simulink model "Expriment_Pose"  (R2014a)
settings: Solver=FixedStepDiscrete  SolverMode=SingleTasking  StartTime=0.0  StopTime=inf  FixedStep=0.01  RelTol=1e-3
PostLoadFcn:
  | h_RPStest = RPStest;
model workspace (MAT data in the model file):
  gtest = 0
undefined symbols (not defined in the file or in its folder): avert, avert_freq_factor, avert_gaze_dirs_chance, avert_gaze_duration_factor, avert_head_frequency_factor, avert_head_speed, BML, BML1, BML2, bmlsL, bmlsM, bodyBusyFlag, clock, emotion_amount_factor, faceBusyFlag, fileID, GAZE_WIN, gazing, mut_freq_factor, mutual_gaze_duration_factor, P, pose_cat_chance, pose_chanc_factor, pose_chance_factor, pose_frequency_factor, pose_lean, pose_lean_flag, pose_speed, pose_twitch, pr, serial, STATE_BEFORE, STATE_GO, STATE_OVER, STATE_READY, Stateflow
libraries: simulink x24, instrumentlib x6, lib_affectiveChar_behavior x2, realtime_pacer_lib x2, lib_affectiveChar_input x1
(part 6 of 7)

== stateflow chart Expriment_Pose/CharacterControl/idlePose_Controller ==
  note: PERSONALITY:
      | -HN: self-touching and object manipulations, non-fluencies rigid posture and minimization of random movements, erect shoulder, cross legs Lean forward tenser
      | -LN:Lean backward reclining, head lean sideway or down
      | -High arousal: self and object adaptors, body tension and random trunk
      | For more info check Burgoon and Koper, 1984.
  note: -Ekman categorized hand poses to Emblems(e.g. hand shrug for helplessness or inability ; thumbs up), illustrators, Regulators, POINTS, Adaptors (self, alter-directed), spontaneousgests, attention-based gests
      | -Picking or squeezing part of the body is aggression against the self or aggression towards others temporarily displaced onto the self;
      | -covering the eye with a hand is relevant to preventing input, avoiding being seen, and shame
      | For more infor refer to Ekman (1972) Hand Movements.
  note: continously unpdate values based on change in valence-arousal
  note: The higher BOREDOMT (treshold), the lower chance of bored pose.
  note: Logically, personality parameters should only get calculated once. Since, here we change the personality dynamically during simulation,we calculate it in each loop.
  note: Problems with priortizing behaviors:
      |     1) When personality change, we want a few adjustments to happen e.g. agent's lean pose changes. The problem is system detects the change and set the flag to 1 and then again goes back to 0. If we dont check in stateflow exactly at that time we dont detect the change. that's why we need another flag that keeps the change till we do the personality based adjustment in behavior.After doing the adjustment we set that flag to zero.
      |     2) We can not use this for tracking if the body is busy at the time. When there is environmnet change agent reacts either by face or body (faceBusyFlag and bodyBusyFlag). We want to stop sending idle BML when they are busy. We need to check if flag is 1 excatly when we want to send the idle body or gaze BML.(if its a few milisec after or before it may not be busy. That's why we need attendChange module to set the flag to 1 for 10 sec after bodyBusy or faceBusy to avoid generating idle behavior in that period.
      |     3)problem also occures when the agent is at the middle of an idle pose/avert and needs to do interactive pose. It causes averted head+smile etc.
  note: Brebner pointed out that frequency of hand movements/gestures was positively correlated with Extraversion [9].
      | Brebner, J. 1985. Personality theory and movement. In B.D. Kirkcaldy (Ed.), Individual differences in movement (pp.
      | 27-41). Lancaster, England: MTP Press Limited.
  note: Riggio suggested that extraverts change their posture more often.
      | Riggio, R., Friedman, H. 1986. Impression formation: The
      | role of expressive behavior. In Journal of Personality and
      | Social Psychology 50(2), 421-427
  state idlePoseGenerate [parallel]
    settings: executionOrder=1
    state stateInit
      entry:STATE_OVER=3;STATE_BEFORE=4;pose_lean_flag=0;
      STATE_READY=7;STATE_GO=1;gameState= 14;
      n=encStr2Arr(' ');bmlsL=[n n n n n];newBmlsL=[n n n n n];
      pose_frequency_factor=20;pose_chance_factor=1;pose_cat_chance=70;
      pose_lean=10; pose_speed=1;pose_lean_flag=0;pose_twitch=0;
    state leanChange
      entry:  pose_lean_flag=0;
      [P,BMLM]=weightshiftTable(pose_lean) ;
      newBmlsM=insertQueue(bmlsM,BMLM);
      bmlsM=newBmlsM;
    state stateRandomPose
      entry: randSlowPose=randArray(:,11);%(1,5)
      interest=BOREDOM_THRESHOLD-boredom;interest=1;
    state stateExtrovertPoseChance
      entry: randPoseChance=randi([0,round(interest*randSlowPose/pose_chance_factor)]);
    note: SLOW
    note: FAST
    note: else
    note: else
    state poseCategoryChance1
      entry: randPR=randArray(:,20);
    state poseCategoryChance2
      entry: randPR=randArray(:,20);
    state poseCategoryChance
      entry: randPR=randArray(:,20);
    note: else
    note: else
    state selfAdaptorPoseCategory
      entry:pose_type=selfAdaptorTypeTable(pose_speed, pose_twitch);
      [P,BMLl]=selfAdaptorTable(randArray(:,pose_type)) ;
      newBmlsL=insertQueueLow(bmlsL,BMLl);
      bmlsL=newBmlsL;%disp(decArr2Str(BMLl));
    state weightshiftPoseCategory
      entry:pose_type=weightShiftTypeTable(pose_speed);
      [P,BMLl]= weightshiftTable(randArray(:,pose_type));
      newBmlsL=insertQueueLow(bmlsL,BMLl);
      bmlsL=newBmlsL;
    (default) -> stateInit
    stateInit -> stateRandomPose
    leanChange -> stateRandomPose : after(1,secs)
    stateRandomPose -> leanChange [order 1] : [pose_lean_flag==1]
    (junction 2) -> stateRandomPose [order 2]
    weightshiftPoseCategory -> stateRandomPose : after(pose_frequency_factor,secs)
    (junction 425) -> stateRandomPose [order 2]
    stateRandomPose -> stateExtrovertPoseChance [order 2]
    selfAdaptorPoseCategory -> stateRandomPose : after(pose_frequency_factor,secs)
    (junction 169) -> stateRandomPose [order 2]
    stateExtrovertPoseChance -> (junction 2) [order 2] : [pose_speed==2]
    stateExtrovertPoseChance -> (junction 425) [order 3] : [pose_speed==1]
    stateExtrovertPoseChance -> (junction 169) [order 1] : [pose_speed==3]
    (junction 425) -> poseCategoryChance2 [order 1] : [[randPoseChance==1]&[ gameState~= STATE_GO]&[ gameState~= STATE_READY]]
    (junction 2) -> poseCategoryChance1 [order 1] : [[randPoseChance==1]&[ gameState~= STATE_GO]&[ gameState~= STATE_READY]]
    (junction 169) -> poseCategoryChance [order 1] : [[randPoseChance==1]&[ gameState~= STATE_GO]&[ gameState~= STATE_READY]]
    poseCategoryChance2 -> poseCategoryChance2 [order 2]
    poseCategoryChance1 -> poseCategoryChance1 [order 2]
    poseCategoryChance -> poseCategoryChance [order 2]
    poseCategoryChance1 -> (junction 344) [order 1] : [bodyBusyFlag~=1]
    poseCategoryChance2 -> (junction 431) [order 1] : [bodyBusyFlag~=1]
    poseCategoryChance -> (junction 340) [order 1] : [bodyBusyFlag~=1]
    (junction 340) -> (junction 212) [order 1] : [randPR<=pose_cat_chance]
    (junction 431) -> (junction 211) [order 2] : [randPR>pose_cat_chance]
    (junction 431) -> (junction 212) [order 1] : [randPR<=pose_cat_chance]
    (junction 344) -> (junction 211) [order 1] : [randPR<=pose_cat_chance]
    (junction 340) -> (junction 211) [order 2] : [randPR>pose_cat_chance ]
    (junction 344) -> (junction 212) [order 2] : [randPR>pose_cat_chance]
    (junction 212) -> weightshiftPoseCategory
    (junction 211) -> selfAdaptorPoseCategory
  note: randSlowPose=randi(1,6)
  note: D10 for animation 8 which is hand on waist may not work with wave etc. Too long!
  note: McNeill's gesture space sectors: the performance space in front of an actor is divided into three gesture space sections: Center-Center (CC), Center (C), and Periphery (P). CC is the central section directly in front of the chest, while subsequent sections (C and P) form spatial layers spreading outwards. low-warmth-low-competence performance consists of gestures mostly in the lower, center P region, while high-warmth-high-competence focuses mostly in the CC and C regions.
  note: LEHN error : more weight shidt
  data: bmlID function_input double; pr function_output double size=1; poseBML function_output double size=[1000,1]; bmlID function_input double; pr function_output double size=1; poseBML function_output double size=[1000,1]; pr function_output double size=1; bmlID function_input double; poseBML function_output double size=[1000,1]; poseSpeed function_input double size=1; shiftType function_output double size=1; poseSpeed function_input double size=1; poseTwitch function_input double size=1; poseType function_output double size=1; bmls function_input double size=[1000,5]; myBML function_input double size=[1000,1]; newBmls function_output double size=[1000,5]; bmls function_input double size=[1000,5]; myBML function_input double size=[1000,1]; newBmls function_output double size=[1000,5]; boredom data_store_memory size=2; BOREDOM_THRESHOLD data_store_memory size=2; randSlowPose data_store_memory size=2; interest data_store_memory size=2; gameState output double size=1; randPoseChance data_store_memory size=1; STATE_OVER data_store_memory size=2; STATE_BEFORE data_store_memory size=2; STATE_READY data_store_memory size=2; inA input double size=1; inE input double size=1; HAPPY data_store_memory size=1 =4; SAD data_store_memory size=1 =4; CONTEMPT data_store_memory size=1 =4; BORED data_store_memory size=1 =4; FRUST data_store_memory size=1 =4; FEAR data_store_memory size=1 =4; IDLE data_store_memory size=1 =4; EXCITE data_store_memory size=1 =4; BML data_store_memory size=[256,1]; P data_store_memory; fileID data_store_memory; STATE_GO data_store_memory; bodyBusyFlag data_store_memory; BMLM local double size=[1000,1]; newBmlsL local double size=[1000,5]; bmlsL data_store_memory; n local; randArray input double size=[1,25]; personality input double size=1; randPR local; pPoseChance local; poseFreq local; leanPose local; inV input double size=1; pPoseChanceP local; poseFreqP local; pCatChance local; catChance local; personalityChange input boolean size=1; bmlsM data_store_memory; BMLl local double size=[1000,1]; newBmlsM local double size=[1000,5]; pChangeFlag local; faceBusyFlag data_store_memory; poseArray input double size=[1, 6]; pose_speed data_store_memory; pose_lean_flag data_store_memory; pose_lean data_store_memory; pose_frequency_factor data_store_memory; pose_chance_factor data_store_memory; pose_cat_chance data_store_memory; pose_change_flag data_store_memory; pose_type local; pose_twitch data_store_memory
  events: secs input RISING_EDGE_EVENT
  function [pr,poseBML]=selfAdaptorTableBilly(bmlID):
    | function [pr,poseBML]=selfAdaptorTableBilly(bmlID)
    | 
    | aVarTruthTableCondition_1 = false;
    | aVarTruthTableCondition_2 = false;
    | aVarTruthTableCondition_3 = false;
    | aVarTruthTableCondition_4 = false;
    | aVarTruthTableCondition_5 = false;
    | aVarTruthTableCondition_6 = false;
    | aVarTruthTableCondition_7 = false;
    | aVarTruthTableCondition_8 = false;
    | aVarTruthTableCondition_9 = false;
    | aVarTruthTableCondition_10 = false;
    | aVarTruthTableCondition_11 = false;
    | aVarTruthTableCondition_12 = false;
    | aVarTruthTableCondition_13 = false;
    | aVarTruthTableCondition_14 = false;
    | aVarTruthTableCondition_15 = false;
    | aVarTruthTableCondition_16 = false;
    | aVarTruthTableCondition_17 = false;
    | aVarTruthTableCondition_18 = false;
    | aVarTruthTableCondition_19 = false;
    | aVarTruthTableCondition_20 = false;
    | 
    | 
    | 
    | aVarTruthTableCondition_1 = logical(bmlID==1);
    | 
    | 
    | aVarTruthTableCondition_2 = logical(bmlID==2);
    | 
    | 
    | aVarTruthTableCondition_3 = logical(bmlID==3);
    | 
    | 
    | aVarTruthTableCondition_4 = logical(bmlID==4);
    | 
    | 
    | aVarTruthTableCondition_5 = logical(bmlID==5);
    | 
    | 
    | aVarTruthTableCondition_6 = logical(bmlID==6);
    | 
    | 
    | aVarTruthTableCondition_7 = logical(bmlID==7);
    | 
    | 
    | aVarTruthTableCondition_8 = logical(bmlID==8);
    | 
    | 
    | aVarTruthTableCondition_9 = logical(bmlID==9);
    | 
    | 
    | aVarTruthTableCondition_10 = logical(bmlID==10);
    | 
    | 
    | aVarTruthTableCondition_11 = logical(bmlID==11);
    | 
    | 
    | aVarTruthTableCondition_12 = logical(bmlID==12);
    | 
    | 
    | aVarTruthTableCondition_13 = logical(bmlID==13);
    | 
    | 
    | aVarTruthTableCondition_14 = logical(bmlID==14);
    | 
    | 
    | aVarTruthTableCondition_15 = logical(bmlID==15);
    | 
    | 
    | aVarTruthTableCondition_16 = logical(bmlID==16);
    | 
    | 
    | aVarTruthTableCondition_17 = logical(bmlID==17);
    | 
    | 
    | aVarTruthTableCondition_18 = logical(bmlID==18);
    | 
    | 
    | aVarTruthTableCondition_19 = logical(bmlID==19);
    | 
    | 
    | aVarTruthTableCondition_20 = logical(bmlID==20);
    | 
    | if (aVarTruthTableCondition_1)
    |     aFcnTruthTableAction_1();
    | elseif (aVarTruthTableCondition_2)
    |     aFcnTruthTableAction_2();
    | elseif (aVarTruthTableCondition_3)
    |     aFcnTruthTableAction_3();
    | elseif (aVarTruthTableCondition_4)
    |     aFcnTruthTableAction_4();
    | elseif (aVarTruthTableCondition_5)
    |     aFcnTruthTableAction_5();
    | elseif (aVarTruthTableCondition_6)
    |     aFcnTruthTableAction_6();
    | elseif (aVarTruthTableCondition_7)
    |     aFcnTruthTableAction_7();
    | elseif (aVarTruthTableCondition_8)
    |     aFcnTruthTableAction_8();
    | elseif (aVarTruthTableCondition_9)
    |     aFcnTruthTableAction_9();
    | elseif (aVarTruthTableCondition_10)
    |     aFcnTruthTableAction_10();
    | elseif (aVarTruthTableCondition_11)
    |     aFcnTruthTableAction_11();
    | elseif (aVarTruthTableCondition_12)
    |     aFcnTruthTableAction_12();
    | elseif (aVarTruthTableCondition_13)
    |     aFcnTruthTableAction_13();
    | elseif (aVarTruthTableCondition_14)
    |     aFcnTruthTableAction_14();
    | elseif (aVarTruthTableCondition_15)
    |     aFcnTruthTableAction_15();
    | elseif (aVarTruthTableCondition_16)
    |     aFcnTruthTableAction_16();
    | elseif (aVarTruthTableCondition_17)
    |     aFcnTruthTableAction_17();
    | elseif (aVarTruthTableCondition_18)
    |     aFcnTruthTableAction_18();
    | elseif (aVarTruthTableCondition_19)
    |     aFcnTruthTableAction_19();
    | elseif (aVarTruthTableCondition_20)
    |     aFcnTruthTableAction_20();
    | else % Default
    |     aFcnTruthTableAction_1();
    | end
    | 
    | function aFcnTruthTableAction_1()
    | 
    | % WeightShiftFast
    | 
    | poseBML=encStr2Arr('<?xml version="1.0" ?><act><bml><animation name="ChrBrad@Idle01_WeightShift01" speed="2" /></bml></act>');pr=3;
    | 
    | function aFcnTruthTableAction_2()
    | 
    | % WeightShift2F
    | 
    | poseBML=encStr2Arr('<?xml version="1.0" ?><act><bml><animation name="ChrBrad@Idle01_WeightShift02" speed="2"/></bml></act>'); pr=3;
    | 
    | function aFcnTruthTableAction_3()
    | 
    | % ShoulderStretchUpDownF
    | 
    | poseBML=encStr2Arr('<?xml version="1.0" ?><act><bml><animation name="ChrBrad@Idle01_ShoulderStretch01" speed="2"/></bml></act>');pr=3;
    | 
    | function aFcnTruthTableAction_4()
    | 
    | % ScratchHeadF
    | 
    | poseBML=encStr2Arr('<?xml version="1.0" ?><act><bml><animation name="ChrBrad@Idle01_ScratchHeadLf01" speed="2"/></bml></act>'); pr=3;
    | 
    | function aFcnTruthTableAction_5()
    | 
    | % scratchtemple(head)F
    | 
    | poseBML=encStr2Arr('<?xml version="1.0" ?><act><bml><animation name="ChrBrad@Idle01_ScratchTempleLf01" speed="2"/></bml></act>'); pr=3;
    | 
    | function aFcnTruthTableAction_6()
    | 
    | % ScratchChestF
    | 
    | poseBML=encStr2Arr('<?xml version="1.0" ?><act><bml><animation name="ChrBrad@Idle01_ScratchChest01" speed="2"/></bml></act>');pr=3;
    | 
    | function aFcnTruthTableAction_7()
    | 
    | % SqueezeHand01F
    | 
    | poseBML=encStr2Arr('<?xml version="1.0" ?><act><bml><animation name="ChrBrad@Idle01_SqueezeHand01" speed="2" /></bml></act>');pr=3;
    | 
    | function aFcnTruthTableAction_8()
    | 
    | % brushCenterF
    | 
    | poseBML=encStr2Arr('<?xml version="1.0" ?><act><bml><gaze angle="10" direction="DOWNLEFT" sbm:joint-range="EYES NECK" sbm:time-hint="2" target="gazeTarget"/><gaze angle="20" direction="DOWNLEFT" sbm:joint-range="EYES" sbm:time-hint="2" target="gazeTarget"/><animation name="../data/ChrBrad/test_idle_brush_center.skm" speed="2"/></bml></act>'); pr=3;
    | 
    | function aFcnTruthTableAction_9()
    | 
    | % lookHandF
    | 
    | poseBML=encStr2Arr('<?xml version="1.0" ?><act><bml><gaze angle="10" direction="DOWNRIGHT" sbm:joint-range="EYES NECK" sbm:time-hint="2" target="gazeTarget"/><gaze angle="20" direction="DOWNRIGHT" sbm:joint-range="EYES" sbm:time-hint="2" target="gazeTarget"/><animation name="../data/ChrBrad/test_idle_hand_look.skm" speed="2"/></bml></act>'); pr=3;
    | 
    | function aFcnTruthTableAction_10()
    | 
    | % TouchHands01Slow-introvert
    | 
    | poseBML=encStr2Arr('<?xml version="1.0" ?><act><bml><animation name="ChrBrad@Idle01_TouchHands01" speed="0.8" /></bml></act>');pr=3;
    | 
    | function aFcnTruthTableAction_11()
    | 
    | % ScratchChestSlow
    | 
    | poseBML=encStr2Arr('<?xml version="1.0" ?><act><bml><animation name="ChrBrad@Idle01_ScratchChest01" speed="1"/></bml></act>');pr=3;
    | 
    | function aFcnTruthTableAction_12()
    | 
    | % WeightShiftSlow
    | 
    | poseBML=encStr2Arr('<?xml version="1.0" ?><act><bml><animation name="ChrBrad@Idle01_WeightShift01" speed="1" /></bml></act>');pr=3;
    | 
    | function aFcnTruthTableAction_13()
    | 
    | % scratchtempleSlow
    | 
    | poseBML=encStr2Arr('<?xml version="1.0" ?><act><bml><animation name="ChrBrad@Idle01_ScratchTempleLf01" speed="1" /></bml></act>');pr=3;
    | 
    | function aFcnTruthTableAction_14()
    | 
    | % SqueezeHandSlow
    | 
    | poseBML=encStr2Arr('<?xml version="1.0" ?><act><bml><animation name="ChrBrad@Idle01_SqueezeHand01" speed="1" /></bml></act>');pr=3;
    | 
    | function aFcnTruthTableAction_15()
    | 
    | % SqueezeHandSlowest
    | 
    | poseBML=encStr2Arr('<?xml version="1.0" ?><act><bml><animation name="ChrBrad@Idle01_SqueezeHand01" speed="0.7" /></bml></act>');pr=3;
    | 
    | function aFcnTruthTableAction_16()
    | 
    | % ShoulderStretchUpDownSlow
    | 
    | poseBML=encStr2Arr('<?xml version="1.0" ?><act><bml><animation name="ChrBrad@Idle01_ShoulderStretch01" speed="1"/></bml></act>');pr=3;
    | 
    | function aFcnTruthTableAction_17()
    | 
    | % WeightShift2Slow
    | 
    | poseBML=encStr2Arr('<?xml version="1.0" ?><act><bml><animation name="ChrBrad@Idle01_WeightShift02" speed="1"/></bml></act>'); pr=3;
    | 
    | function aFcnTruthTableAction_18()
    | 
    | % brushArmS
    | 
    | poseBML=encStr2Arr('<?xml version="1.0" ?><act><bml><gaze angle="20" direction="DOWNLEFT" sbm:joint-range="EYES NECK" sbm:time-hint="1" target="gazeTarget"/><gaze angle="30" direction="DOWNLEFT" sbm:joint-range="EYES" sbm:time-hint="1" target="gazeTarget"/><animation name="../data/ChrBrad/test_idle_brush.skm" speed="1"/></bml></act>'); pr=3;
    | 
    | function aFcnTruthTableAction_19()
    | 
    | % brushChestS
    | 
    | poseBML=encStr2Arr('<?xml version="1.0" ?><act><bml><gaze angle="10" direction="DOWNLEFT" sbm:joint-range="EYES NECK" sbm:time-hint="1" target="gazeTarget"/><gaze angle="20" direction="DOWNLEFT" sbm:joint-range="EYES" sbm:time-hint="1" target="gazeTarget"/><animation name="../data/ChrBrad/test_idle_brush_center.skm" speed="1"/></bml></act>'); pr=3;
    | 
    | function aFcnTruthTableAction_20()
    | 
    | % gazeAtHandS
    | 
    | poseBML=encStr2Arr('<?xml version="1.0" ?><act><bml><gaze angle="10" direction="DOWNRIGHT" sbm:joint-range="EYES NECK" sbm:time-hint="1" target="gazeTarget"/><gaze angle="20" direction="DOWNRIGHT" sbm:joint-range="EYES" sbm:time-hint="1" target="gazeTarget"/><animation name="../data/ChrBrad/test_idle_hand_look.skm" speed="1"/></bml></act>'); pr=3;
  function [pr,poseBML]=selfAdaptorTable(bmlID):
    | function [pr,poseBML]=selfAdaptorTable(bmlID)
    | 
    | aVarTruthTableCondition_1 = false;
    | aVarTruthTableCondition_2 = false;
    | aVarTruthTableCondition_3 = false;
    | aVarTruthTableCondition_4 = false;
    | aVarTruthTableCondition_5 = false;
    | aVarTruthTableCondition_6 = false;
    | aVarTruthTableCondition_7 = false;
    | aVarTruthTableCondition_8 = false;
    | aVarTruthTableCondition_9 = false;
    | aVarTruthTableCondition_10 = false;
    | aVarTruthTableCondition_11 = false;
    | aVarTruthTableCondition_12 = false;
    | aVarTruthTableCondition_13 = false;
    | 
    | 
    | 
    | aVarTruthTableCondition_1 = logical(bmlID==1);
    | 
    | 
    | aVarTruthTableCondition_2 = logical(bmlID==2);
    | 
    | 
    | aVarTruthTableCondition_3 = logical(bmlID==3);
    | 
    | 
    | aVarTruthTableCondition_4 = logical(bmlID==4);
    | 
    | 
    | aVarTruthTableCondition_5 = logical(bmlID==5);
    | 
    | 
    | aVarTruthTableCondition_6 = logical(bmlID==6);
    | 
    | 
    | aVarTruthTableCondition_7 = logical(bmlID==7);
    | 
    | 
    | aVarTruthTableCondition_8 = logical(bmlID==8);
    | 
    | 
    | aVarTruthTableCondition_9 = logical(bmlID==9);
    | 
    | 
    | aVarTruthTableCondition_10 = logical(bmlID==10);
    | 
    | 
    | aVarTruthTableCondition_11 = logical(bmlID==11);
    | 
    | 
    | aVarTruthTableCondition_12 = logical(bmlID==12);
    | 
    | 
    | aVarTruthTableCondition_13 = logical(bmlID==13);
    | 
    | if (aVarTruthTableCondition_1)
    |     aFcnTruthTableAction_1();
    | elseif (aVarTruthTableCondition_2)
    |     aFcnTruthTableAction_2();
    | elseif (aVarTruthTableCondition_3)
    |     aFcnTruthTableAction_3();
    | elseif (aVarTruthTableCondition_4)
    |     aFcnTruthTableAction_4();
    | elseif (aVarTruthTableCondition_5)
    |     aFcnTruthTableAction_5();
    | elseif (aVarTruthTableCondition_6)
    |     aFcnTruthTableAction_6();
    | elseif (aVarTruthTableCondition_7)
    |     aFcnTruthTableAction_7();
    | elseif (aVarTruthTableCondition_8)
    |     aFcnTruthTableAction_8();
    | elseif (aVarTruthTableCondition_9)
    |     aFcnTruthTableAction_9();
    | elseif (aVarTruthTableCondition_10)
    |     aFcnTruthTableAction_10();
    | elseif (aVarTruthTableCondition_11)
    |     aFcnTruthTableAction_11();
    | elseif (aVarTruthTableCondition_12)
    |     aFcnTruthTableAction_12();
    | elseif (aVarTruthTableCondition_13)
    |     aFcnTruthTableAction_13();
    | else % Default
    |     aFcnTruthTableAction_1();
    | end
    | 
    | function aFcnTruthTableAction_1()
    | 
    | % ScratchHeadFast
    | 
    | poseBML=encStr2Arr('<?xml version="1.0" ?><act><bml><animation name="ChrBrad@Idle01_ScratchHeadLf01" speed="1.5"/></bml></act>'); pr=3;
    | 
    | function aFcnTruthTableAction_2()
    | 
    | % scratchtemple(head)F
    | 
    | poseBML=encStr2Arr('<?xml version="1.0" ?><act><bml><animation name="ChrBrad@Idle01_ScratchTempleLf01" speed="1.5"/></bml></act>'); pr=3;
    | 
    | function aFcnTruthTableAction_3()
    | 
    | % ScratchChestF
    | 
    | poseBML=encStr2Arr('<?xml version="1.0" ?><act><bml><animation name="ChrBrad@Idle01_ScratchChest01" speed="1.5"/></bml></act>');pr=3;
    | 
    | function aFcnTruthTableAction_4()
    | 
    | % TouchHands01F
    | 
    | poseBML=encStr2Arr('<?xml version="1.0" ?><act><bml><animation name="ChrBrad@Idle01_TouchHands01" speed="1.5" /></bml></act>');pr=3;
    | 
    | function aFcnTruthTableAction_5()
    | 
    | % SqueezeHand01F
    | 
    | poseBML=encStr2Arr('<?xml version="1.0" ?><act><bml><animation name="ChrBrad@Idle01_SqueezeHand01"  speed="1.5"/></bml></act>');pr=3;
    | 
    | function aFcnTruthTableAction_6()
    | 
    | % twitchF
    | 
    | poseBML=encStr2Arr('<?xml version="1.0" ?><act><bml><animation name="ChrBrad@Idle01_ShoulderStretch01" speed="3"/></bml></act>');pr=3;
    | 
    | function aFcnTruthTableAction_7()
    | 
    | % TouchHands01Slow-introvert
    | 
    | poseBML=encStr2Arr('<?xml version="1.0" ?><act><bml><animation name="ChrBrad@Idle01_TouchHands01" speed="0.8" /></bml></act>');pr=3;
    | 
    | function aFcnTruthTableAction_8()
    | 
    | % ScratchChestSlow
    | 
    | poseBML=encStr2Arr('<?xml version="1.0" ?><act><bml><animation name="ChrBrad@Idle01_ScratchChest01" speed="0.6"/></bml></act>');pr=3;
    | 
    | function aFcnTruthTableAction_9()
    | 
    | % scratchtempleSlow
    | 
    | poseBML=encStr2Arr('<?xml version="1.0" ?><act><bml><animation name="ChrBrad@Idle01_ScratchTempleLf01" speed="0.6" /></bml></act>');pr=3;
    | 
    | function aFcnTruthTableAction_10()
    | 
    | % SqueezeHandSlow
    | 
    | poseBML=encStr2Arr('<?xml version="1.0" ?><act><bml><animation name="ChrBrad@Idle01_SqueezeHand01" speed="0.6" /></bml></act>');pr=3;
    | 
    | function aFcnTruthTableAction_11()
    | 
    | % ScratchHeadS
    | 
    | poseBML=encStr2Arr('<?xml version="1.0" ?><act><bml><animation name="ChrBrad@Idle01_ScratchHeadLf01" speed="0.6"/></bml></act>'); pr=3;
    | 
    | function aFcnTruthTableAction_12()
    | 
    | % SqueezeHandS2
    | 
    | poseBML=encStr2Arr('<?xml version="1.0" ?><act><bml><animation name="ChrBrad@Idle01_SqueezeHand01" speed="0.5" /></bml></act>');pr=3;
    | 
    | function aFcnTruthTableAction_13()
    | 
    | % twitchS
    | 
    | poseBML=encStr2Arr('<?xml version="1.0" ?><act><bml><animation name="ChrBrad@Idle01_ShoulderStretch01" speed="2"/></bml></act>');pr=3;
  function [pr,poseBML]=weightshiftTable(bmlID):
    | function [pr,poseBML]=weightshiftTable(bmlID)
    | 
    | aVarTruthTableCondition_1 = false;
    | aVarTruthTableCondition_2 = false;
    | aVarTruthTableCondition_3 = false;
    | aVarTruthTableCondition_4 = false;
    | aVarTruthTableCondition_5 = false;
    | aVarTruthTableCondition_6 = false;
    | aVarTruthTableCondition_7 = false;
    | aVarTruthTableCondition_8 = false;
    | aVarTruthTableCondition_9 = false;
    | aVarTruthTableCondition_10 = false;
    | aVarTruthTableCondition_11 = false;
    | 
    | 
    | 
    | aVarTruthTableCondition_1 = logical(bmlID==1);
    | 
    | 
    | aVarTruthTableCondition_2 = logical(bmlID==2);
    | 
    | 
    | aVarTruthTableCondition_3 = logical(bmlID==3);
    | 
    | 
    | aVarTruthTableCondition_4 = logical(bmlID==4);
    | 
    | 
    | aVarTruthTableCondition_5 = logical(bmlID==5);
    | 
    | 
    | aVarTruthTableCondition_6 = logical(bmlID==6);
    | 
    | 
    | aVarTruthTableCondition_7 = logical(bmlID==7);
    | 
    | 
    | aVarTruthTableCondition_8 = logical(bmlID==8);
    | 
    | 
    | aVarTruthTableCondition_9 = logical(bmlID==9);
    | 
    | 
    | aVarTruthTableCondition_10 = logical(bmlID==10);
    | 
    | 
    | aVarTruthTableCondition_11 = logical(bmlID==11);
    | 
    | if (aVarTruthTableCondition_1)
    |     aFcnTruthTableAction_1();
    | elseif (aVarTruthTableCondition_2)
    |     aFcnTruthTableAction_2();
    | elseif (aVarTruthTableCondition_3)
    |     aFcnTruthTableAction_3();
    | elseif (aVarTruthTableCondition_4)
    |     aFcnTruthTableAction_4();
    | elseif (aVarTruthTableCondition_5)
    |     aFcnTruthTableAction_5();
    | elseif (aVarTruthTableCondition_6)
    |     aFcnTruthTableAction_6();
    | elseif (aVarTruthTableCondition_7)
    |     aFcnTruthTableAction_7();
    | elseif (aVarTruthTableCondition_8)
    |     aFcnTruthTableAction_8();
    | elseif (aVarTruthTableCondition_9)
    |     aFcnTruthTableAction_9();
    | elseif (aVarTruthTableCondition_10)
    |     aFcnTruthTableAction_10();
    | elseif (aVarTruthTableCondition_11)
    |     aFcnTruthTableAction_11();
    | else % Default
    |     aFcnTruthTableAction_1();
    | end
    | 
    | function aFcnTruthTableAction_1()
    | 
    | % ShoulderStretchUpDownFast
    | 
    | poseBML=encStr2Arr('<?xml version="1.0" ?><act><bml><animation name="ChrBrad@Idle01_ShoulderStretch01" speed="1.5"/></bml></act>');pr=3;
    | 
    | function aFcnTruthTableAction_2()
    | 
    | % WeightShiftFast
    | 
    | poseBML=encStr2Arr('<?xml version="1.0" ?><act><bml><animation name="ChrBrad@Idle01_WeightShift01" speed="1.7"/></bml></act>');pr=3;;
    | 
    | function aFcnTruthTableAction_3()
    | 
    | % WeightShift2Fast
    | 
    | poseBML=encStr2Arr('<?xml version="1.0" ?><act><bml><animation name="ChrBrad@Idle01_WeightShift01"  speed="1.7"/></bml></act>');pr=3;;
    | 
    | function aFcnTruthTableAction_4()
    | 
    | % Idle01_ToIdle02Fast
    | 
    | poseBML=encStr2Arr('<?xml version="1.0" ?><act><bml><animation name="ChrBrad@Idle01_ToIdle02" speed="1.7"/></bml></act>');pr=4;
    | 
    | function aFcnTruthTableAction_5()
    | 
    | % armStretchF
    | 
    | poseBML=encStr2Arr('<?xml version="1.0" ?><act><bml><animation name="ChrBrad@Idle01_ArmStretch01" speed="1.5"/></bml></act>');pr=3;
    | 
    | function aFcnTruthTableAction_6()
    | 
    | % Idle01_ToIdle02Slow
    | 
    | poseBML=encStr2Arr('<?xml version="1.0" ?><act><bml><animation name="ChrBrad@Idle01_ToIdle02" speed="0.6"/></bml></act>');pr=4;
    | 
    | function aFcnTruthTableAction_7()
    | 
    | % WeightShift2Slow
    | 
    | poseBML=encStr2Arr('<?xml version="1.0" ?><act><bml><animation name="ChrBrad@Idle01_WeightShift02" speed="0.6"/></bml></act>'); pr=3;
    | 
    | function aFcnTruthTableAction_8()
    | 
    | % WeightShiftSlow
    | 
    | poseBML=encStr2Arr('<?xml version="1.0" ?><act><bml><animation name="ChrBrad@Idle01_WeightShift01" speed="0.6" /></bml></act>');pr=3;
    | 
    | function aFcnTruthTableAction_9()
    | 
    | % ShoulderStretchUpDownSlow
    | 
    | poseBML=encStr2Arr('<?xml version="1.0" ?><act><bml><animation name="ChrBrad@Idle01_ShoulderStretch01" speed="0.6"/></bml></act>');pr=3;
    | 
    | function aFcnTruthTableAction_10()
    | 
    | % extrovertLeanBack
    | 
    | poseBML=encStr2Arr('<?xml version="1.0" ?><act><bml><gaze angle="3" direction="UP" sbm:joint-range="HEAD CHEST" sbm:time-hint="2" target="gazeTarget"/></bml></act>'); pr=3;
    | 
    | function aFcnTruthTableAction_11()
    | 
    | % introvertLeanFW
    | 
    | poseBML=encStr2Arr('<?xml version="1.0" ?><act><bml><gaze angle="3" direction="DOWN" sbm:joint-range="HEAD CHEST" sbm:time-hint="2" target="gazeTarget"/></bml></act>'); pr=3;
    | 
    | function aFcnTruthTableAction_12()
    | 
    | % NotUsed
    | 
    | poseBML=encStr2Arr('<?xml version="1.0" ?><act><bml><animation name="ChrBrad@Idle01_ToIdle02" speed="2"/></bml></act>');pr=4;
    | 
    | function aFcnTruthTableAction_13()
    | 
    | % notUsed2
    | 
    | poseBML=encStr2Arr('<?xml version="1.0" ?><act><bml><animation name="ChrBrad@Idle01_ToIdle03" start="0" ready="1" stroke="2" stroke_end="3" relax="18" end="20" /></bml></act>');pr=4;
  function shiftType = weightShiftTypeTable(poseSpeed):
    | function shiftType = weightShiftTypeTable(poseSpeed)
    | 
    | aVarTruthTableCondition_1 = false;
    | aVarTruthTableCondition_2 = false;
    | aVarTruthTableCondition_3 = false;
    | 
    | 
    | % FastWS
    | 
    | aVarTruthTableCondition_1 = logical([[poseSpeed==2]]);
    | 
    | % SlowWS
    | 
    | aVarTruthTableCondition_2 = logical([[poseSpeed==1]]);
    | 
    | % NormalWS
    | 
    | aVarTruthTableCondition_3 = logical([[poseSpeed==0]]);
    | 
    | if (aVarTruthTableCondition_1)
    |     aFcnTruthTableAction_1();
    | elseif (aVarTruthTableCondition_2)
    |     aFcnTruthTableAction_2();
    | elseif (aVarTruthTableCondition_3)
    |     aFcnTruthTableAction_3();
    | else % Default
    |     aFcnTruthTableAction_1();
    | end
    | 
    | function aFcnTruthTableAction_1()
    | 
    | % FastWS
    | 
    | shiftType=21;
    | 
    | function aFcnTruthTableAction_2()
    | 
    | % SlowWS
    | 
    | shiftType=22;
    | 
    | function aFcnTruthTableAction_3()
    | 
    | % normalWS
    | 
    | shiftType=22;
  function poseType = selfAdaptorTypeTable(poseSpeed, poseTwitch):
    | function poseType = selfAdaptorTypeTable(poseSpeed, poseTwitch)
    | 
    | aVarTruthTableCondition_1 = false;
    | aVarTruthTableCondition_2 = false;
    | aVarTruthTableCondition_3 = false;
    | aVarTruthTableCondition_4 = false;
    | 
    | 
    | % Fast-Twitch
    | 
    | aVarTruthTableCondition_1 = logical([[poseSpeed==2]&[poseTwitch==1]]);
    | 
    | % Slow-Twitch
    | 
    | aVarTruthTableCondition_2 = logical([[poseSpeed==1]&[poseTwitch==1]]);
    | 
    | % Fast-NoTwitch
    | 
    | aVarTruthTableCondition_3 = logical([[poseSpeed==2]&[poseTwitch==0]]);
    | 
    | % Slow-NoTwitch
    | 
    | aVarTruthTableCondition_4 = logical([[poseSpeed==1]&[poseTwitch==0]]);
    | 
    | if (aVarTruthTableCondition_1)
    |     aFcnTruthTableAction_1();
    | elseif (aVarTruthTableCondition_2)
    |     aFcnTruthTableAction_2();
    | elseif (aVarTruthTableCondition_3)
    |     aFcnTruthTableAction_3();
    | elseif (aVarTruthTableCondition_4)
    |     aFcnTruthTableAction_4();
    | else % Default
    |     aFcnTruthTableAction_2();
    | end
    | 
    | function aFcnTruthTableAction_1()
    | 
    | % FastTwitch
    | 
    | poseType=13;
    | 
    | function aFcnTruthTableAction_2()
    | 
    | % SlowTwitch
    | 
    | poseType=14;
    | 
    | function aFcnTruthTableAction_3()
    | 
    | % FastNoTwitch
    | 
    | poseType=23;
    | 
    | function aFcnTruthTableAction_4()
    | 
    | % SlowNoTwitch
    | 
    | poseType=24;
  function newBmls =insertQueueLow(bmls,myBML):
    | function newBmls =insertQueueLow(bmls,myBML)
    |     full=1;
    |     t=encStr2Arr(' ');
    |     newBmls=[t t t t t];
    |     for i = 1:5
    |         if (isequal(bmls(:,i),t))
    |             %add to end of the queue where its empty
    |             bmls(:,i)=myBML;
    |             full=0;
    |             break
    |         end
    |     end
    |     if(full~=0)
    |             %if queue full, shift all elements to left which removes the first one, then add to end
    |             bmls(:,1)= bmls(:,2);
    |             bmls(:,2)= bmls(:,3);
    |             bmls(:,3)= bmls(:,4);
    |             bmls(:,5)=myBML;
    |     end
    |     newBmls=bmls;
  function newBmls =insertQueue(bmls,myBML):
    | function newBmls =insertQueue(bmls,myBML)
    |     full=1;
    |     t=encStr2Arr(' ');
    |     newBmls=[t t t t t];
    |     for i = 1:5
    |         if (isequal(bmls(:,i),t))
    |             %add to end of the queue where its empty
    |             bmls(:,i)=myBML;
    |             full=0;
    |             break
    |         end
    |     end
    |     if(full~=0)
    |             %if queue full, shift all elements to left which removes the first one, then add to end
    |             bmls(:,1)= bmls(:,2);
    |             bmls(:,2)= bmls(:,3);
    |             bmls(:,3)= bmls(:,4);
    |             bmls(:,5)=myBML;
    |     end
    |     newBmls=bmls;

== matlab function Expriment_Pose/moveFWTable ==
  data: z input; y output
function y = fcn(z)

aVarTruthTableCondition_1 = false;
aVarTruthTableCondition_2 = false;
aVarTruthTableCondition_3 = false;
aVarTruthTableCondition_4 = false;


% too far

aVarTruthTableCondition_1 = logical(z >= 220);

% too close

aVarTruthTableCondition_2 = logical(z < 150 && z~=0);

% properSpace

aVarTruthTableCondition_3 = logical(z>=150 && z<220);

% no value

aVarTruthTableCondition_4 = logical(z==0);

if (aVarTruthTableCondition_1)
    aFcnTruthTableAction_1();
elseif (aVarTruthTableCondition_2)
    aFcnTruthTableAction_2();
elseif (aVarTruthTableCondition_3)
    aFcnTruthTableAction_3();
elseif (aVarTruthTableCondition_4)
    aFcnTruthTableAction_4();
else % Default
    aFcnTruthTableAction_4();
end

function aFcnTruthTableAction_1()

% too far

y = 2;

function aFcnTruthTableAction_2()

% too close

y = 1;

function aFcnTruthTableAction_3()

% properSpace

y = 0;

function aFcnTruthTableAction_4()

% no value

y = 3;

== matlab function Expriment_Pose/gazeTable ==
  data: x input; y output
function y = fcn(x)

aVarTruthTableCondition_1 = false;
aVarTruthTableCondition_2 = false;


% moved left

aVarTruthTableCondition_1 = logical(x > 50);

% moved right

aVarTruthTableCondition_2 = logical(x < -50);

if (aVarTruthTableCondition_1)
    aFcnTruthTableAction_1();
elseif (aVarTruthTableCondition_2)
    aFcnTruthTableAction_2();
else % Default
    aFcnTruthTableAction_3();
end

function aFcnTruthTableAction_1()

% moved left

y = 1;

function aFcnTruthTableAction_2()

% moved right

y = 2;

function aFcnTruthTableAction_3()

% proper place

y = 0;

== stateflow chart Expriment_Pose/CharacterControl/personalSpace_Controller ==
  state stateInit
    entry: gameState=14;
    TOO_CLOSE=1;TOO_FAR=2;NEUTRAL=0;
    farBuffer=0;closeBuffer=0;neutralBuffer=0;position=1;
    n=encStr2Arr(' ');bmlsM=[n n n n n];newBmlsM=[n n n n n];
    bmlsL=[n n n n n];newBmlsL=[n n n n n];
  note: Problem:
      | Sometimes locomotion BML is sent (visible in the vhmsgYarpRelais) but it is not running. Also smartbody shows duplicate msg id error. It seems that when too many BMLs are sent to smartbody some of them have same IDs.
  state wait
  note: if avert not 1
  state gazeSurprized
    entry: [P,BMLM]=walkInvadingTable(5) ;
    closeBuffer=closeBuffer+1;
    newBmlsM=insertQueue(bmlsM,BMLM);
    bmlsM=newBmlsM;
  state doIt3Times
    entry: position=2;
    closeBuffer=0;
  note: User is too close!
  state headNeuralGazeCamera
    entry: [P,BMLM]=walkInvadingTable(4) ;
    newBmlsM=insertQueue(bmlsM,BMLM);
    bmlsM=newBmlsM;
  state stateWalkBack
    entry:  [P,BMLM]=walkInvadingTable(2);
    newBmlsM=insertQueue(bmlsM,BMLM);  bmlsM=newBmlsM;
    closeBuffer=closeBuffer+1;
  state browUp
    entry: [P,BMLM]=walkInvadingTable(8) ;
    neutralBuffer=neutralBuffer+1;
    newBmlsM=insertQueue(bmlsM,BMLM);
    bmlsM=newBmlsM;
  state doIt3Times1
    entry: position=1;
    neutralBuffer=0;
  note: EXE ORDER IMPORTANT
  state checkUserCoord
  note: correct: [zChange==1]{position=0;}
  state idle
    entry: [P,BMLM]=walkInvadingTable(1);
    newBmlsM=insertQueue(bmlsM,BMLM);
    bmlsM=newBmlsM;
    neutralBuffer=neutralBuffer+1;
  note: User is in the middle!
  state wait2
  state leanFW
    entry: [P,BMLM]=walkInvadingTable(6) ;
    farBuffer=farBuffer+1;
    newBmlsM=insertQueue(bmlsM,BMLM);
    bmlsM=newBmlsM;
  state doIt3Times2
    entry: position=3;
    farBuffer=0;
  note: Problem:
      | We dont know where smatbody is standing (z pos). If smartbody does not run the locomotion BML sent for any reason (too many BMLs), we want to send locomodation BML again after a while to make sure the personal space is correct. On the other hand, we dont want the module to keep sending move bmls.
  state walkFW
    entry:  [P,BMLM]=walkInvadingTable(3) ;
    newBmlsM=insertQueue(bmlsM,BMLM);  bmlsM=newBmlsM;
    farBuffer=farBuffer+1;
  note: User is too far!
  state leanNeutral
    entry:  [P,BMLM]=walkInvadingTable(7) ;
    newBmlsM=insertQueue(bmlsM,BMLM); bmlsM=newBmlsM;
  (default) -> stateInit
  stateInit -> (junction 2)
  wait -> (junction 2)
  (junction 2) -> headNeuralGazeCamera [order 1] : [avert==1]
  (junction 2) -> checkUserCoord [order 2]
  idle -> wait [order 2] : after(5,secs)
  walkFW -> wait [order 2] : after(5,secs)
  stateWalkBack -> wait [order 2] : after(5,secs)
  doIt3Times1 -> wait : after(5,secs)
  doIt3Times2 -> wait : after(5,secs)
  doIt3Times -> wait : after(5,secs)
  checkUserCoord -> (junction 89) [order 3] : [[distance==TOO_CLOSE]&[position~=2]]
  (junction 89) -> gazeSurprized [order 2] : [closeBuffer<2]
  (junction 89) -> stateWalkBack [order 1] : [closeBuffer>=2]
  stateWalkBack -> doIt3Times [order 1] : [closeBuffer==5]
  gazeSurprized -> checkUserCoord
  headNeuralGazeCamera -> checkUserCoord
  checkUserCoord -> (junction 92) [order 2] : [[distance==NEUTRAL]&[position~=1]]
  (junction 92) -> browUp [order 1] : [neutralBuffer<2]
  wait2 -> checkUserCoord [order 1] : [zChange==1]{position=0;}
  idle -> doIt3Times1 [order 1] : [neutralBuffer==5]
  browUp -> checkUserCoord
  (junction 92) -> idle [order 2] : [neutralBuffer>=2]
  wait2 -> checkUserCoord [order 2] : [zChange~=1]
  checkUserCoord -> wait2 [order 4] : after(20,secs)
  checkUserCoord -> (junction 87) [order 1] : [[distance==TOO_FAR]&[position~=3]]
  leanFW -> checkUserCoord
  (junction 87) -> leanFW [order 2] : [farBuffer<2]
  walkFW -> doIt3Times2 [order 1] : [farBuffer==5]
  (junction 87) -> leanNeutral [order 1] : [farBuffer>=2]
  leanNeutral -> walkFW : after(2,secs)
  data: bmls function_input double size=[1000,5]; myBML function_input double size=[1000,1]; newBmls function_output double size=[1000,5]; p function_output double size=1; bmlID function_input double size=1; poseBML function_output double size=[1000,1]; bmls function_input double size=[1000,5]; myBML function_input double size=[1000,1]; newBmls function_output double size=[1000,5]; gameState output double size=1; STATE_READY data_store_memory size=1; STATE_OVER data_store_memory size=1; distance input double size=1; STATE_BEFORE data_store_memory size=1; BML1 data_store_memory size=[256,1]; P data_store_memory; pr data_store_memory; fileID data_store_memory; neutralBuffer local; closeBuffer local; NEUTRAL local; TOO_FAR local; TOO_CLOSE local; farBuffer local; zChange input; position local; avert data_store_memory; newBmlsM local double size=[1000,5]; bmlsM data_store_memory; BMLM local double size=[1000,1]; BMLL local double size=[1000,1]; newBmlsL local double size=[1000,5]; bmlsL data_store_memory; n local
  events: secs input RISING_EDGE_EVENT
  function newBmls =insertQueueLow(bmls,myBML):
    | function newBmls =insertQueueLow(bmls,myBML)
    |     full=1;
    |     t=encStr2Arr(' ');
    |     newBmls=[t t t t t];
    |     for i = 1:5
    |         if (isequal(bmls(:,i),t))
    |             %add to end of the queue where its empty
    |             bmls(:,i)=myBML;
    |             full=0;
    |             break
    |         end
    |     end
    |     if(full~=0)
    |             %if queue full, shift all elements to left which removes the first one, then add to end
    |             bmls(:,1)= bmls(:,2);
    |             bmls(:,2)= bmls(:,3);
    |             bmls(:,3)= bmls(:,4);
    |             bmls(:,5)=myBML;
    |     end
    |     newBmls=bmls;
  function [p,poseBML]=walkInvadingTable(bmlID):
    | function [p,poseBML]=walkInvadingTable(bmlID)
    | 
    | aVarTruthTableCondition_1 = false;
    | aVarTruthTableCondition_2 = false;
    | aVarTruthTableCondition_3 = false;
    | aVarTruthTableCondition_4 = false;
    | aVarTruthTableCondition_5 = false;
    | aVarTruthTableCondition_6 = false;
    | aVarTruthTableCondition_7 = false;
    | aVarTruthTableCondition_8 = false;
    | 
    | 
    | % n
    | 
    | aVarTruthTableCondition_1 = logical(bmlID==1);
    | 
    | % b
    | 
    | aVarTruthTableCondition_2 = logical(bmlID==2);
    | 
    | % f
    | 
    | aVarTruthTableCondition_3 = logical(bmlID==3);
    | 
    | % HN
    | 
    | aVarTruthTableCondition_4 = logical(bmlID==4);
    | 
    | % surprizeGaze
    | 
    | aVarTruthTableCondition_5 = logical(bmlID==5);
    | 
    | % leanFw
    | 
    | aVarTruthTableCondition_6 = logical(bmlID==6);
    | 
    | % leanNeutral
    | 
    | aVarTruthTableCondition_7 = logical(bmlID==7);
    | 
    | % browUp
    | 
    | aVarTruthTableCondition_8 = logical(bmlID==8);
    | 
    | if (aVarTruthTableCondition_1)
    |     aFcnTruthTableAction_1();
    | elseif (aVarTruthTableCondition_2)
    |     aFcnTruthTableAction_2();
    | elseif (aVarTruthTableCondition_3)
    |     aFcnTruthTableAction_3();
    | elseif (aVarTruthTableCondition_4)
    |     aFcnTruthTableAction_4();
    | elseif (aVarTruthTableCondition_5)
    |     aFcnTruthTableAction_5();
    | elseif (aVarTruthTableCondition_6)
    |     aFcnTruthTableAction_6();
    | elseif (aVarTruthTableCondition_7)
    |     aFcnTruthTableAction_7();
    | elseif (aVarTruthTableCondition_8)
    |     aFcnTruthTableAction_8();
    | else % Default
    |     aFcnTruthTableAction_1();
    | end
    | 
    | function aFcnTruthTableAction_1()
    | 
    | % Neutral
    | 
    | poseBML=encStr2Arr( '<?xml version="1.0" ?><act><bml><locomotion manner="walk" facing="gazeTarget"  sbm:accel="0.5" sbm:scootaccel="50" target="0 0"/></bml></act>');p=1;
    | 
    | function aFcnTruthTableAction_2()
    | 
    | % Back
    | 
    | poseBML=encStr2Arr( '<?xml version="1.0" ?><act><bml><locomotion manner="walk"  sbm:accel="0.5" sbm:scootaccel="50" facing="gazeTarget" target="0 -0.6"/></bml></act>');p=1;
    | 
    | function aFcnTruthTableAction_3()
    | 
    | % Forward
    | 
    | poseBML=encStr2Arr( '<?xml version="1.0" ?><act><bml><locomotion manner="walk" facing="gazeTarget"  sbm:accel="0.5" sbm:scootaccel="50" target="0 0.6"/></bml></act>');p=1;
    | 
    | function aFcnTruthTableAction_4()
    | 
    | % NeutralHead
    | 
    | poseBML=encStr2Arr('<?xml version="1.0" ?><act><bml><gaze target="gazeTarget" sbm:joint-range="EYES NECK" sbm:time-hint="1.5"/></bml></act>');p=1;
    | 
    | function aFcnTruthTableAction_5()
    | 
    | % surprisedGaze
    | 
    | poseBML=encStr2Arr('<?xml version="1.0" ?><act><bml><face type="FACS" start="0" end="5" side="BOTH" au="5" relax="3" amount="0.5"/><face type="FACS" start="0" end="5" side="BOTH" au="2" relax="3" amount="0.5"/></bml></act>');p=1;
    | 
    | function aFcnTruthTableAction_6()
    | 
    | % leanFW
    | 
    | poseBML=encStr2Arr('<?xml version="1.0" ?><act><bml><gaze angle="5" direction="DOWN" sbm:joint-range="HEAD BACK" sbm:time-hint="2" target="gazeTarget"/></bml></act>');p=1;
    | 
    | function aFcnTruthTableAction_7()
    | 
    | % leanNeutral
    | 
    | poseBML=encStr2Arr('<?xml version="1.0" ?><act><bml><gaze sbm:time-hint="2" target="gazeTarget"/></bml></act>');p=1;
    | 
    | function aFcnTruthTableAction_8()
    | 
    | % browUp
    | 
    | poseBML=encStr2Arr('<?xml version="1.0" ?><act><bml><face au="2" end="5" ready="1" relax="4" side="BOTH" start="0" stroke="3" type="facs"/></bml></act>');p=1;
  function newBmls =insertQueue(bmls,myBML):
    | function newBmls =insertQueue(bmls,myBML)
    |     full=1;
    |     t=encStr2Arr(' ');
    |     newBmls=[t t t t t];
    |     for i = 1:5
    |         if (isequal(bmls(:,i),t))
    |             %add to end of the queue where its empty
    |             bmls(:,i)=myBML;
    |             full=0;
    |             break
    |         end
    |     end
    |     if(full~=0)
    |             %if queue full, shift all elements to left which removes the first one, then add to end
    |             bmls(:,1)= bmls(:,2);
    |             bmls(:,2)= bmls(:,3);
    |             bmls(:,3)= bmls(:,4);
    |             bmls(:,5)=myBML;
    |     end
    |     newBmls=bmls;
